simulink model "modeSelector"  (R2023a)
settings: Solver=ode4  StartTime=0.0  StopTime=10.0  FixedStep=dt  RelTol=1e-3
undefined symbols (not defined in the file): enableGNC
settings Model: Creator=hugobuurmeijer  LastModifiedBy=ndelurgio

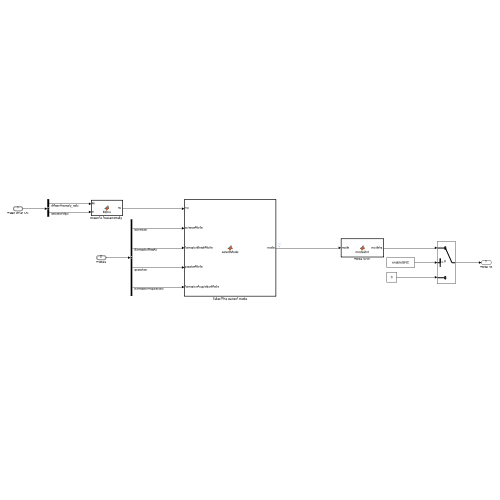
[thumbnail: Simulink's stored preview of the top-level diagram]
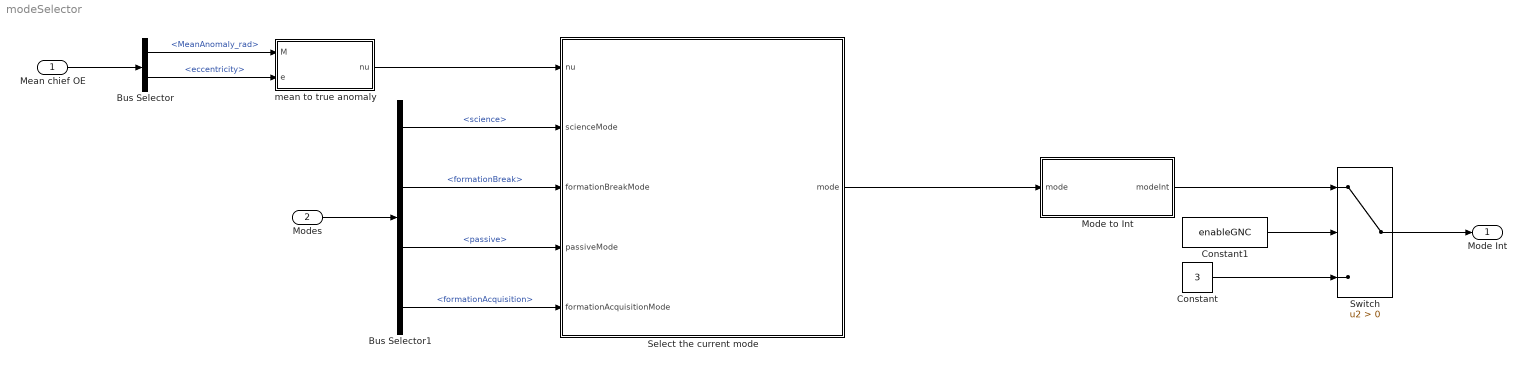
== system modeSelector ==
  Mean chief OE : Inport  OutDataTypeStr=Bus: meanOrbitElements
  Modes : Inport  Port=2  OutDataTypeStr=Bus: modes
  Bus Selector : BusSelector  OutputSignals=MeanAnomaly_rad,eccentricity
  Bus Selector1 : BusSelector  OutputSignals=science,formationBreak,passive,formationAcquisition
  Constant : Constant  Value=3
  Constant1 : Constant  Value=enableGNC
  Mode to Int : MATLAB Function  TreatAsAtomicUnit=on
  Select the current mode : MATLAB Function  TreatAsAtomicUnit=on
  Switch : Switch  Criteria=u2 > Threshold  SaturateOnIntegerOverflow=off  InputSameDT=off
  "mean to true anomaly " : MATLAB Function  TreatAsAtomicUnit=on
  Mode Int : Outport
  wires:
  "mean to true anomaly "/1(nu) -> Select the current mode/1(nu)
  Bus Selector/2 -> "mean to true anomaly "/2(e)  "<eccentricity>"
  Mean chief OE/1 -> Bus Selector/1
  Bus Selector/1 -> "mean to true anomaly "/1(M)  "<MeanAnomaly_rad>"
  Modes/1 -> Bus Selector1/1
  Bus Selector1/1 -> Select the current mode/2(scienceMode)  "<science>"
  Bus Selector1/2 -> Select the current mode/3(formationBreakMode)  "<formationBreak>"
  Bus Selector1/3 -> Select the current mode/4(passiveMode)  "<passive>"
  Bus Selector1/4 -> Select the current mode/5(formationAcquisitionMode)  "<formationAcquisition>"
  Select the current mode/1(mode) -> Mode to Int/1(mode)
  Mode to Int/1(modeInt) -> Switch/1
  Constant/1 -> Switch/3
  Constant1/1 -> Switch/2
  Switch/1 -> Mode Int/1

== matlab function modeSelector/Select the current mode ==
  data: nu input; mode output; scienceMode input; formationBreakMode input; passiveMode input; formationAcquisitionMode input
function mode = selectMode(nu, scienceMode, formationBreakMode, passiveMode, formationAcquisitionMode)

mode = selectMode(nu, scienceMode, formationBreakMode, passiveMode, formationAcquisitionMode);

end

== matlab function modeSelector/mean to true anomaly  ==
  data: M input; nu output; e input
function nu = M2nu(M, e)

nu = M2nu(M, e);

end

== matlab function modeSelector/Mode to Int ==
  data: mode input; modeInt output
function modeInt = mode2int(mode)
modeInt = mode2int(mode);
end
